simulink model "normal_openloop"  (R2018b)
settings: Solver=FixedStepAuto  StartTime=0.0  StopTime=100  FixedStep=0.1  RelTol=1e-3
settings Model: Creator=afsha  LastModifiedBy=afsha

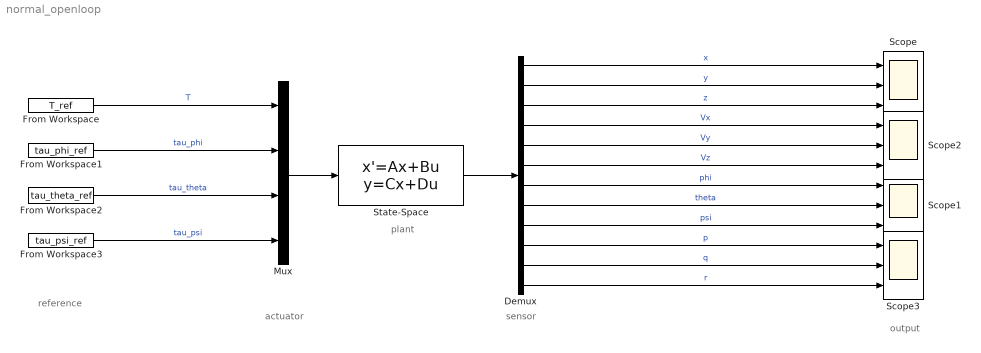
== system normal_openloop ==
  note: output
  note: sensor
  note: actuator
  note: plant
  note: reference
  Demux : Demux  Outputs=12
  From Workspace : FromWorkspace  VariableName=T_ref  SampleTime=0
  From Workspace1 : FromWorkspace  VariableName=tau_phi_ref  SampleTime=0
  From Workspace2 : FromWorkspace  VariableName=tau_theta_ref  SampleTime=0
  From Workspace3 : FromWorkspace  VariableName=tau_psi_ref  SampleTime=0
  Mux : Mux
  Scope{,1..3} (4 alike) : Scope  NumInputPorts=3
  State-Space : StateSpace  A=|  B=|  C=eye(12)  D=zeros(12, 4)  InitialCondition=[0 0 0 0 0 0 0 0 0 0 0 0]  ContinuousStateAttributes={'x', 'y', 'z', 'Vx', 'Vy', 'Vz', 'phi', 'theta', 'psi', 'p', 'q', 'r'}
      A=|
      | [0 0 0 1 0 0 0 0 0 0 0 0;
      |  0 0 0 0 1 0 0 0 0 0 0 0;
      |  0 0 0 0 0 1 0 0 0 0 0 0;
      |  0 0 0 0 0 0 0 -g 0 0 0 0;
      |  0 0 0 0 0 0 g 0 0 0 0 0;
      |  0 0 0 0 0 0 0 0 0 0 0 0;
      |  0 0 0 0 0 0 0 0 0 1 0 0;
      |  0 0 0 0 0 0 0 0 0 0 1 0;
      |  0 0 0 0 0 0 0 0 0 0 0 1;
      |  0 0 0 0 0 0 0 0 0 0 0 0;
      |  0 0 0 0 0 0 0 0 0 0 0 0;
      |  0 0 0 0 0 0 0 0 0 0 0 0]
      B=|
      | [0 0 0 0;
      |       0 0 0 0;
      |       0 0 0 0;
      |       0 0 0 0;
      |       0 0 0 0;
      |       1/m  0 0 0;
      |       0 0 0 0;
      |       0 0 0 0;
      |       0 0 0 0;
      |       0 1/Jx 0 0;
      |       0 0 1/Jy 0;
      |       0 0 0 1/Jz]
  wires:
  State-Space/1 -> Demux/1
  Mux/1 -> State-Space/1
  Demux/1 -> Scope/1  "x"
  Demux/2 -> Scope/2  "y"
  Demux/3 -> Scope/3  "z"
  Demux/7 -> Scope1/1  "phi"
  Demux/8 -> Scope1/2  "theta"
  Demux/9 -> Scope1/3  "psi"
  Demux/4 -> Scope2/1  "Vx"
  Demux/5 -> Scope2/2  "Vy"
  Demux/6 -> Scope2/3  "Vz"
  Demux/10 -> Scope3/1  "p"
  Demux/11 -> Scope3/2  "q"
  Demux/12 -> Scope3/3  "r"
  From Workspace3/1 -> Mux/4  "tau_psi"
  From Workspace/1 -> Mux/1  "T"
  From Workspace1/1 -> Mux/2  "tau_phi"
  From Workspace2/1 -> Mux/3  "tau_theta"
